simulink model "ALU"  (R2018a)
settings: Solver=VariableStepAuto  StartTime=0.0  StopTime=10.0  RelTol=1e-3
settings Model: Creator=midog  LastModifiedBy=midog

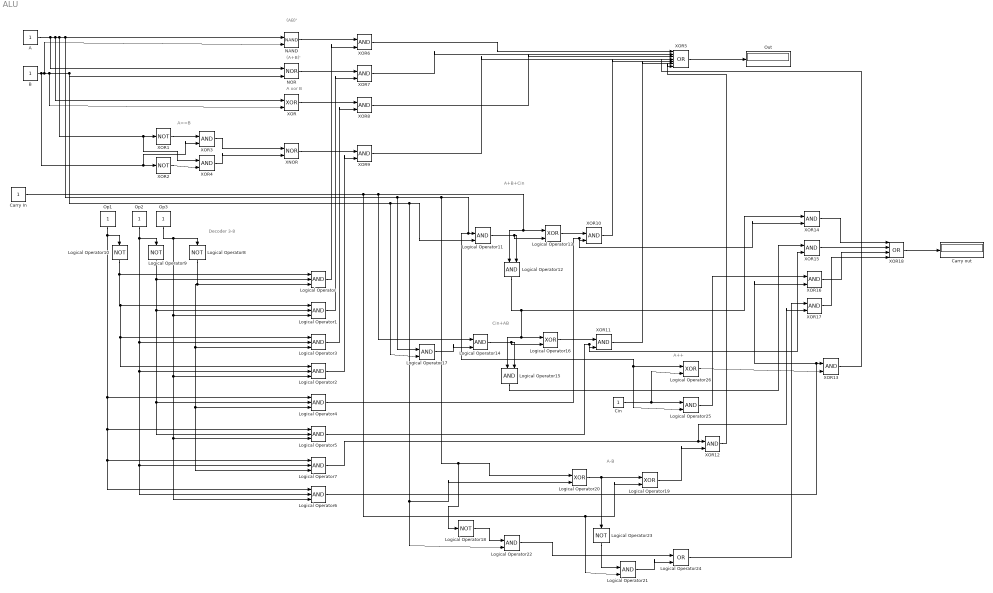
== system ALU ==
  note: A==B
  note: (AB)'
  note: (A+B)'
  note: A xor B
  note: A+B+Cin
  note: Cin+AB
  note: A-B
  note: A++
  note: Decoder 3-8
  A : Constant
  B : Constant
  "Carry In " : Constant
  Carry out : Display
  Cin : Constant
  Logical Operator{,1..7} (8 alike) : Logic  Inputs=3  IconShape=distinctive  AllPortsSameDT=off  OutDataTypeStr=boolean
  Logical Operator10 : Logic  Operator=NOT  Inputs=1  IconShape=distinctive  AllPortsSameDT=off  OutDataTypeStr=boolean
  Logical Operator{11..12,14..15,17,21..22,25} (8 alike) : Logic  IconShape=distinctive  AllPortsSameDT=off  OutDataTypeStr=boolean
  Logical Operator{13,16,19..20,26} (5 alike) : Logic  Operator=XOR  IconShape=distinctive  AllPortsSameDT=off  OutDataTypeStr=boolean
  Logical Operator18 : Logic  Operator=NOT  IconShape=distinctive  AllPortsSameDT=off  OutDataTypeStr=boolean
  Logical Operator23 : Logic  Operator=NOT  IconShape=distinctive  AllPortsSameDT=off  OutDataTypeStr=boolean
  Logical Operator24 : Logic  Operator=OR  IconShape=distinctive  AllPortsSameDT=off  OutDataTypeStr=boolean
  Logical Operator8 : Logic  Operator=NOT  Inputs=1  IconShape=distinctive  AllPortsSameDT=off  OutDataTypeStr=boolean
  Logical Operator9 : Logic  Operator=NOT  Inputs=1  IconShape=distinctive  AllPortsSameDT=off  OutDataTypeStr=boolean
  NAND : Logic  Operator=NAND  IconShape=distinctive  AllPortsSameDT=off  OutDataTypeStr=boolean
  NOR : Logic  Operator=NOR  IconShape=distinctive  AllPortsSameDT=off  OutDataTypeStr=boolean
  "Op1 " : Constant
  Op2 : Constant
  Op3 : Constant
  Out : Display
  XNOR : Logic  Operator=NOR  IconShape=distinctive  AllPortsSameDT=off  OutDataTypeStr=boolean
  XOR : Logic  Operator=XOR  IconShape=distinctive  AllPortsSameDT=off  OutDataTypeStr=boolean
  XOR1 : Logic  Operator=NOT  IconShape=distinctive  AllPortsSameDT=off  OutDataTypeStr=boolean
  XOR{3..4,6..17} (14 alike) : Logic  IconShape=distinctive  AllPortsSameDT=off  OutDataTypeStr=boolean
  XOR18 : Logic  Operator=OR  Inputs=4  IconShape=distinctive  AllPortsSameDT=off  OutDataTypeStr=boolean
  XOR2 : Logic  Operator=NOT  IconShape=distinctive  AllPortsSameDT=off  OutDataTypeStr=boolean
  XOR5 : Logic  Operator=OR  Inputs=8  IconShape=distinctive  AllPortsSameDT=off  OutDataTypeStr=boolean
  wires:
  Op3/1 -> Logical Operator8/1, Logical Operator1/3, Logical Operator2/3, Logical Operator6/3, Logical Operator5/3
  Logical Operator8/1 -> Logical Operator3/3, Logical Operator7/3, Logical Operator4/3, Logical Operator/3
  Op2/1 -> Logical Operator3/2, Logical Operator2/2, Logical Operator6/2, Logical Operator7/2, Logical Operator9/1
  Logical Operator9/1 -> Logical Operator/2, Logical Operator1/2, Logical Operator5/2, Logical Operator4/2
  "Op1 "/1 -> Logical Operator4/1, Logical Operator5/1, Logical Operator7/1, Logical Operator6/1, Logical Operator10/1
  Logical Operator10/1 -> Logical Operator2/1, Logical Operator3/1, Logical Operator1/1, Logical Operator/1
  Logical Operator/1 -> XOR6/2
  Logical Operator1/1 -> XOR7/2
  Logical Operator3/1 -> XOR8/2
  Logical Operator2/1 -> XOR9/2
  Logical Operator5/1 -> XOR15/2, XOR11/2
  XOR3/1 -> XNOR/1
  XOR4/1 -> XNOR/2
  XOR2/1 -> XOR4/2
  XOR1/1 -> XOR3/1
  NAND/1 -> XOR6/1
  NOR/1 -> XOR7/1
  XOR/1 -> XOR8/1
  XNOR/1 -> XOR9/1
  Logical Operator11/1 -> Logical Operator13/2, Logical Operator12/2
  XOR6/1 -> XOR5/1
  XOR7/1 -> XOR5/2
  XOR8/1 -> XOR5/3
  XOR9/1 -> XOR5/4
  Logical Operator12/1 -> XOR14/1, Logical Operator15/1, Logical Operator16/1
  Logical Operator14/1 -> Logical Operator16/2, Logical Operator15/2
  Logical Operator17/1 -> Logical Operator14/2
  Logical Operator13/1 -> XOR10/1
  Logical Operator16/1 -> XOR11/1
  Logical Operator4/1 -> XOR14/2, XOR10/2
  XOR10/1 -> XOR5/5
  XOR11/1 -> XOR5/6
  Logical Operator21/1 -> Logical Operator24/2
  "Carry In "/1 -> Logical Operator21/2, Logical Operator19/2, Logical Operator14/1, Logical Operator12/1, Logical Operator13/1
  Logical Operator22/1 -> Logical Operator24/1
  Logical Operator18/1 -> Logical Operator22/1
  B/1 -> XOR3/2, XOR2/1, NAND/2, XOR/2, Logical Operator17/2, Logical Operator20/2, Logical Operator22/2, Logical Operator11/2, NOR/2
  Logical Operator23/1 -> Logical Operator21/1
  Logical Operator20/1 -> Logical Operator23/1, Logical Operator19/1
  Logical Operator19/1 -> XOR12/2
  Logical Operator7/1 -> XOR17/2, XOR12/1
  XOR12/1 -> XOR5/7
  Cin/1 -> Logical Operator26/2, Logical Operator25/1
  A/1 -> NOR/1, XOR/1, Logical Operator17/1, Logical Operator18/1, Logical Operator20/1, Logical Operator25/2, Logical Operator26/1, Logical Operator11/1, NAND/1, XOR4/1, XOR1/1
  Logical Operator26/1 -> XOR13/2
  Logical Operator6/1 -> XOR16/2, XOR13/1
  XOR13/1 -> XOR5/8
  XOR5/1 -> Out/1
  Logical Operator15/1 -> XOR15/1
  Logical Operator24/1 -> XOR17/1
  Logical Operator25/1 -> XOR16/1
  XOR14/1 -> XOR18/1
  XOR15/1 -> XOR18/2
  XOR16/1 -> XOR18/3
  XOR17/1 -> XOR18/4
  XOR18/1 -> Carry out/1
